simulink model "ex1"  (R2023b)
settings: Solver=VariableStepAuto  StartTime=0.0  StopTime=10.0  RelTol=1e-3
settings Model: Creator=jamesvaughan  LastModifiedBy=jamesvaughan

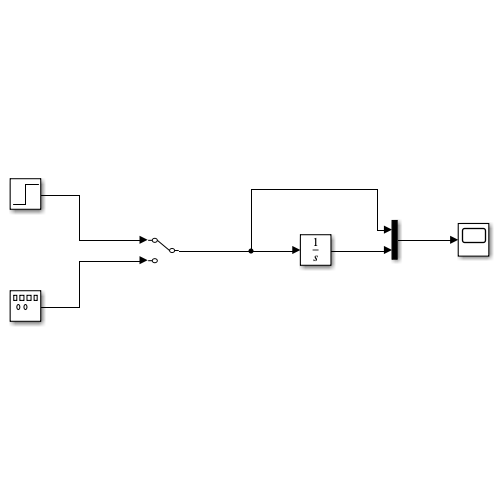
[thumbnail: Simulink's stored preview of the top-level diagram]
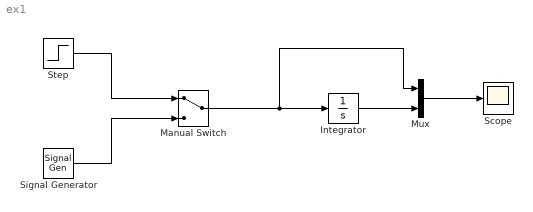
== system ex1 ==
  Integrator : Integrator
  Manual Switch : ManualSwitch
  Mux : Mux  Inputs=2
  Scope : Scope
  Signal Generator : SignalGenerator  Units=rad/sec
  Step : Step  SampleTime=0
  wires:
  Step/1 -> Manual Switch/1
  Signal Generator/1 -> Manual Switch/2
  Manual Switch/1 -> Mux/1, Integrator/1
  Integrator/1 -> Mux/2
  Mux/1 -> Scope/1
